simulink model "untitled"  (R2023a)
settings: Solver=VariableStepAuto  StartTime=0.0  StopTime=10.0  RelTol=1e-3
settings Model: Creator=User  LastModifiedBy=User

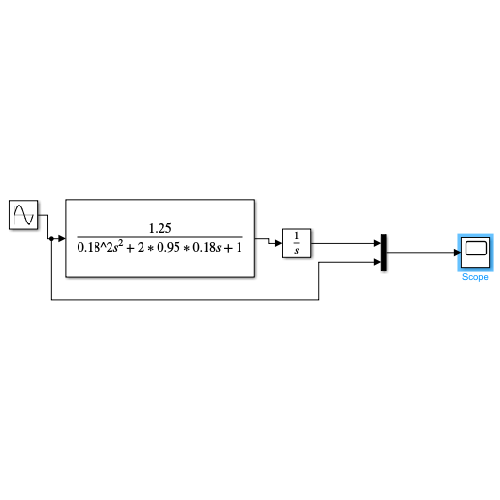
[thumbnail: Simulink's stored preview of the top-level diagram]
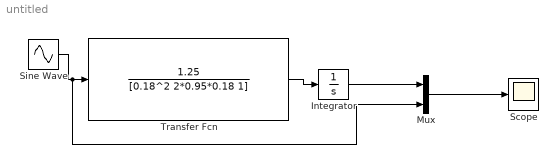
== system untitled ==
  Integrator : Integrator
  Mux : Mux  Inputs=2
  Scope : Scope
  Sine Wave : Sin  SampleTime=0
  Transfer Fcn : TransferFcn  Numerator=[1.25]  Denominator=[0.18^2 2*0.95*0.18 1]
  wires:
  Transfer Fcn/1 -> Integrator/1
  Integrator/1 -> Mux/1
  Sine Wave/1 -> Mux/2, Transfer Fcn/1
  Mux/1 -> Scope/1
